simulink model "ysw7_10"  (R2014a)
settings: Solver=ode15s  StartTime=0.0  StopTime=1  RelTol=1e-3
libraries: powerlib x4
settings Model: Creator=Administrator  LastModifiedBy=Administrator

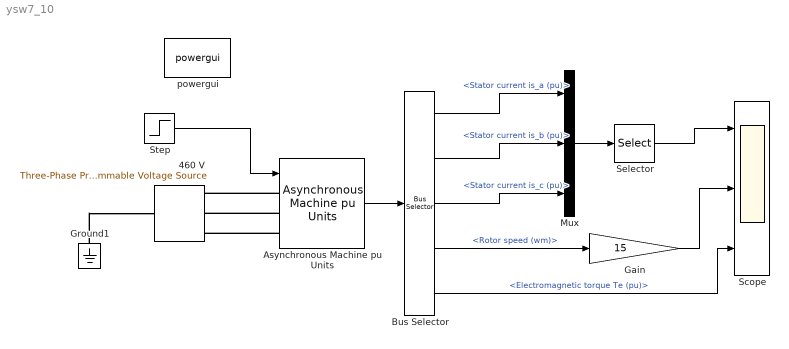
== system ysw7_10 ==
  460 V : powerlib/Electrical Sources/Three-Phase Programmable Voltage Source  PositiveSequence="[460  0 60]"  VariationEntity=None  VariationType=Step  VariationTypeAlt=Step  VariationStep=0.5  VariationRate=10  VariationMagnitude=0.3  VariationFrequency=2  VariationTiming=[1 2]  VariationPhaseA=off  Amplitudes=[1 0.8 1.2 1.0]  TimeValues=[0 0.1 0.15 0.2]  HarmonicGeneration=off  HarmonicA=[3 0.2 -25 0]  HarmonicB=[2 0.15 35 2]  Timing="[0.05  3]"  BusType=swing  Pref=0  Qref=0  Qmin=-inf  Qmax=inf
  Asynchronous Machine pu Units : powerlib/Machines/Asynchronous Machine pu Units  PresetModel=No  MechanicalLoad=Torque Tm  ShowDetailedParameters=on  RotorType=Squirrel-cage  ReferenceFrame=Rotor  Units=pu  MeasurementBus=off  NominalParameters=[10000 380 50]  Stator=[0.458 2.578e-03]  Rotor=[0.349 0.333e-02]  Cage1=[0.01909 0.0397]  Cage2=[0.01909 0.0397]  Lm=0.088  Mechanical=[0.6 0.0 2]  PolePairs=2  InitialConditions="[ 1,0   0,0,0   0,0,0 ]"  SimulateSaturation=off  Saturation="[0.212,0.4201,0.8125,1.0979,1.4799,2.2457,3.2586,4.5763,6.4763 ;   0.5,0.7,0.9,1,1.1,1.2 ,1.3,1.4,1.5]"  LoadFlowParameters=0  TsPowergui=0  TsBlock=-1  IterativeModel=Trapezoidal non iterative  Pmec=0
  Bus Selector : BusSelector  OutputSignals=Stator measurements.Stator current is_a (pu),Stator measurements.Stator current is_b (pu),Stator measurements.Stator current is_c (pu),Mechanical.Rotor speed (wm),Mechanical.Electromagnetic torque Te (pu)
  Gain : Gain  Gain=15
  Ground1 : powerlib/Elements/Ground  LConnTagsString=a
  Mux : Mux  Inputs=3
  Scope : Scope  NumInputPorts=3
      settings: YMin=-5~-5~-5  YMax=5~5~5
  Selector : Selector  InputPortWidth=3  Indices=[1]
  Step : Step  Time=0.2  Before=67.7642  After=100  SampleTime=0
  powergui : powerlib/powergui  Priority=1  SimulationMode=Continuous  SolverType=Tustin  SampleTime=50e-6  frequency=60  SPID=off  DisableSnubberDevices=off  DisableRonSwitches=off  DisableVfSwitches=off  SwTol=0  Interpol=off  DisplayEquations=off  Ts=0  methode=off  frequencyindice=50  Pbase=100e6  ErrMax=1e-4  Iterations=50  UnitsV=kV  UnitsW=MW  FunctionMessages=off  echomessages=off  HookPort=off  EnableUseOfTLC=off  x0status=blocks  RestoreLinks=warning  ResistiveCurrentMeasurement=off  Frange=[0:2:500]  Ylog=off  Xlog=on  ShowGrid=off  save=off  variable=ZData  structure=0  ZoomFFT=off  StartTime=0.0  cycles=1  DisplayStyle=1  fundamental=60  FreqAxis=off  MaxFrequency=1000  frequencyindicesteady=1  RmsSteady=1  display=off
  wires:
  Step/1 -> Asynchronous Machine pu Units/1
  Asynchronous Machine pu Units/1 -> Bus Selector/1
  Bus Selector/1 -> Mux/1  "<Stator current is_a (pu)>"
  Bus Selector/2 -> Mux/2  "<Stator current is_b (pu)>"
  Bus Selector/3 -> Mux/3  "<Stator current is_c (pu)>"
  Mux/1 -> Selector/1
  Selector/1 -> Scope/1
  Bus Selector/4 -> Gain/1  "<Rotor speed (wm)>"
  Gain/1 -> Scope/2
  Bus Selector/5 -> Scope/3  "<Electromagnetic torque Te (pu)>"
  connections:
  Asynchronous Machine pu Units/LConn2 -- 460 V/RConn2
  Asynchronous Machine pu Units/LConn1 -- 460 V/RConn1
  Asynchronous Machine pu Units/LConn3 -- 460 V/RConn3
  Ground1/LConn1 -- 460 V/LConn1
